simulink model "PSA_isa_velocity_control"  (R2020b)
settings: Solver=VariableStepAuto  StartTime=0.0  StopTime=40  RelTol=1e-3
values from neighbouring files (symbols this model uses):
  Kd = 1.2    [PSA_init.m]
  Kp = 1.5    [PSA_init.m]
  Lambda1 = 0.2    [PSA_init.m]
  tau1 = 0.7    [PSA_init.m]
undefined symbols (not defined in the file or in its folder): sigbuilder_block, x0
libraries: pid_lib x1
settings Model: Creator=anime  LastModifiedBy=anime

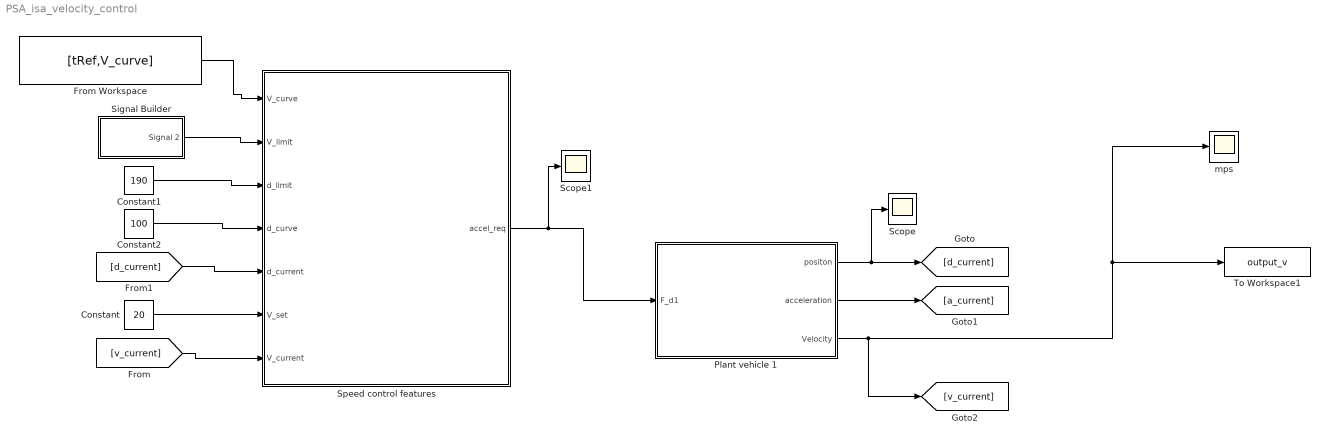
== system PSA_isa_velocity_control ==
  Constant : Constant  Value=20
  Constant1 : Constant  Value=190
  Constant2 : Constant  Value=100
  From Workspace : FromWorkspace  VariableName=[tRef,V_curve]  SampleTime=0.1
  Plant vehicle 1 : Subsystem
  Scope : Scope
  Scope1 : Scope
  Signal Builder : Subsystem  Tag=STV Subsys  LoadFcn=sigbuilder_block('load');  StartFcn=sigbuilder_block('start');  StopFcn=sigbuilder_block('stop');  ClipboardFcn=sigbuilder_block('clipboard');  mask(Sigbuilder block){tuvar=[0:10]}
      mask help: Simulink:masks:SigbuilderBlock_MD
      mask init:
      | if ~strcmp(get_param(bdroot(gcbh),'SimulationStatus'),'stopped') tuvar = sigbuilder_block('maskInit'); end
      settings: CopyFcn=sigbuilder_block('copy');  DeleteFcn=sigbuilder_block('delete');  ModelCloseFcn=sigbuilder_block('modelClose');  PreSaveFcn=sigbuilder_block('preSave');  PauseFcn=sigbuilder_block('pause');  ContinueFcn=sigbuilder_block('continue');  NameChangeFcn=sigbuilder_block('namechange');  OpenFcn=sigbuilder_block('open',[235.2 67.2 550.8 400.2 ]);  CloseFcn=sigbuilder_block('close');
      mask Display: plot(0, 0, 100, 100,[2, 2, 32, 32, 2], [68, 8, 8, 68, 68],[32, 2], [38, 38], [32, 19, 2],[53, 60, 44], [32, 17, 17, 2],[16, 16, 31, 31]);txt = getActiveGroup(gcbh);text(2, 100, txt,'verticalAlignment', 'top');
  Speed control features : Subsystem
  To Workspace1 : ToWorkspace  VariableName=output_v  SaveFormat=Timeseries  SampleTime=-1
  mps : Scope
  wires:
  Plant vehicle 1/3(Velocity) -> [v_current], mps/1, To Workspace1/1
  Plant vehicle 1/1(positon) -> Scope/1, [d_current]
  Plant vehicle 1/2(acceleration) -> [a_current]
  Speed control features/1(accel_req) -> Scope1/1, Plant vehicle 1/1(F_d1)
  [v_current] -> Speed control features/7(V_current)
  [d_current] -> Speed control features/5(d_current)
  Constant/1 -> Speed control features/6(V_set)
  Signal Builder/1(Signal 2) -> Speed control features/2(V_limit)
  Constant1/1 -> Speed control features/3("d_limit ")
  Constant2/1 -> Speed control features/4(d_curve)
  From Workspace/1 -> Speed control features/1(V_curve)

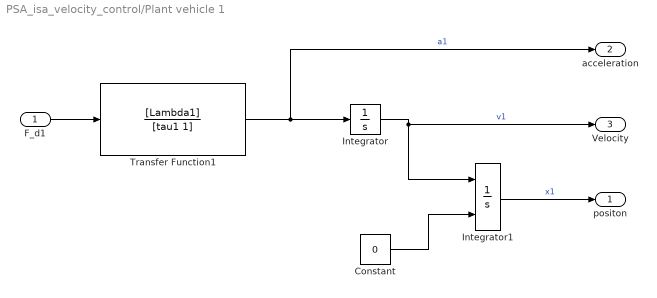
== system PSA_isa_velocity_control/Plant vehicle 1 ==
  F_d1 : Inport
  Constant : Constant  Value=0
  Integrator : Integrator  InitialCondition=3
  Integrator1 : Integrator  InitialConditionSource=external  InitialCondition=x0
  Transfer Function1 : TransferFcn  Numerator=[Lambda1]  Denominator=[tau1 1]
  positon : Outport
  acceleration : Outport  Port=2
  Velocity : Outport  Port=3
  wires:
  F_d1/1 -> Transfer Function1/1
  Transfer Function1/1 -> acceleration/1, Integrator/1  "a1"
  Integrator/1 -> Velocity/1, Integrator1/1  "v1"
  Constant/1 -> Integrator1/2
  Integrator1/1 -> positon/1  "x1"

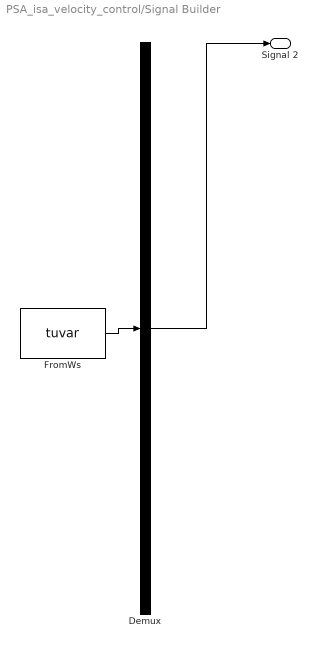
== system PSA_isa_velocity_control/Signal Builder ==
  Demux : Demux  Tag=STV Demux  Outputs=1
      settings: DisplayOption=none
  FromWs : FromWorkspace  Tag=STV FromWs  VariableName=tuvar
      SigBuilderData=|
      | common.afterFinalStr = 'Extrapolate'
      | common.sampleTime = 0
      | dataSet.timeRange = [0 40]
      | dataSet.name = 'Group 1'
      | sbobj.Groups.Name = 'Group 1'
      | sbobj.Groups.Signals.Name = 'Signal 2'
      | sbobj.Groups.Signals.XData = [0 25.2 25.2 40]
      | sbobj.Groups.Signals.YData = [11.11 11.11 16.667 16.667]
      | sbobj.Groups.TimeRange = [0 40]
  Signal 2 : Outport  Tag=STV Outport
  wires:
  FromWs/1 -> Demux/1
  Demux/1 -> Signal 2/1

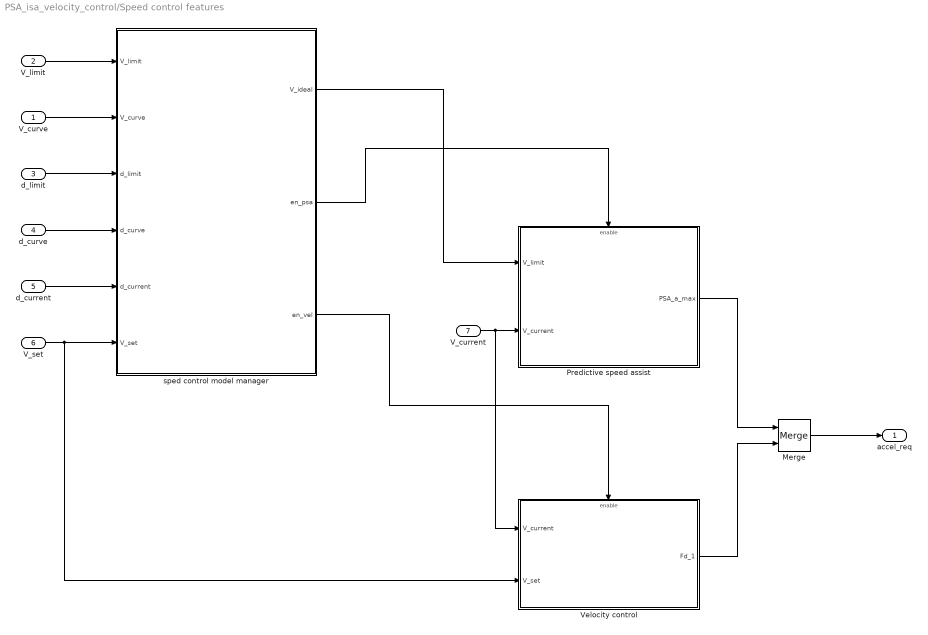
== system PSA_isa_velocity_control/Speed control features ==
  V_curve : Inport
  V_limit : Inport  Port=2
  "d_limit " : Inport  Port=3
  d_curve : Inport  Port=4
  d_current : Inport  Port=5
  V_set : Inport  Port=6
  V_current : Inport  Port=7
  Merge : Merge
  Predictive speed assist : Subsystem
  Velocity control : Subsystem
  sped control model manager : Subsystem
  accel_req : Outport
  wires:
  V_limit/1 -> sped control model manager/1(V_limit)
  "d_limit "/1 -> sped control model manager/3("d_limit ")
  d_curve/1 -> sped control model manager/4(d_curve)
  d_current/1 -> sped control model manager/5(d_current)
  V_set/1 -> Velocity control/2(V_set), sped control model manager/6(V_set)
  sped control model manager/3(en_vel) -> Velocity control/Enable
  sped control model manager/2(en_psa) -> Predictive speed assist/Enable
  sped control model manager/1(V_ideal) -> Predictive speed assist/1(V_limit)
  V_current/1 -> Velocity control/1(V_current), Predictive speed assist/2(V_current)
  Predictive speed assist/1(PSA_a_max) -> Merge/1
  Velocity control/1(Fd_1) -> Merge/2
  Merge/1 -> accel_req/1
  V_curve/1 -> sped control model manager/2(V_curve)

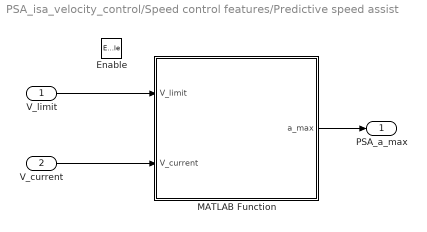
== system PSA_isa_velocity_control/Speed control features/Predictive speed assist ==
  V_limit : Inport
  V_current : Inport  Port=2
  Enable : EnablePort
  MATLAB Function : MATLAB Function  TreatAsAtomicUnit=on
  PSA_a_max : Outport
  wires:
  V_limit/1 -> MATLAB Function/1(V_limit)
  V_current/1 -> MATLAB Function/2(V_current)
  MATLAB Function/1(a_max) -> PSA_a_max/1

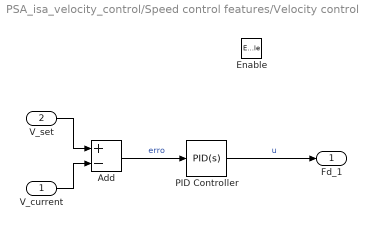
== system PSA_isa_velocity_control/Speed control features/Velocity control ==
  V_current : Inport
  V_set : Inport  Port=2
  Enable : EnablePort
  Add : Sum  Inputs=+-
  PID Controller : pid_lib/PID Controller  Controller=PID  Form=Parallel  TimeDomain=Continuous-time  UseExternalTs=off  SampleTime=-1  IntegratorMethod=Forward Euler  FilterMethod=Forward Euler  ControllerParametersSource=internal  P=Kp  I=0  D=Kd  UseFilter=on  N=100  TunerSelectOption=Transfer Function Based (PID Tuner App)  InitialConditionSource=internal  InitialConditionForIntegrator=0  InitialConditionForFilter=0  DifferentiatorICPrevScaledInput=0  ExternalReset=none  TrackingMode=off  Kt=1  LimitOutput=off  SatLimitsSource=internal  UpperSaturationLimit=inf  LowerSaturationLimit=-inf  LinearizeAsGain=on  AntiWindupMode=none  Kb=1  POutMin=[]  POutMax=[]  IOutMin=[]  IOutMax=[]  DOutMin=[]  DOutMax=[]  NOutMin=[]  NOutMax=[]  SumOutMin=[]  SumOutMax=[]  SaturationOutMin=[]  SaturationOutMax=[]  PParamMin=[]  PParamMax=[]  IParamMin=[]  IParamMax=[]  DParamMin=[]  DParamMax=[]  NParamMin=[]  NParamMax=[]  KbParamMin=[]  KbParamMax=[]  KtParamMin=[]  KtParamMax=[]  KbOutMin=[]  KbOutMax=[]  KtOutMin=[]  KtOutMax=[]  IntegratorOutMin=[]  IntegratorOutMax=[]  FilterOutMin=[]  FilterOutMax=[]  SumI1OutMin=[]  SumI1OutMax=[]  SumI2OutMin=[]  SumI2OutMax=[]  SumI3OutMin=[]  SumI3OutMax=[]  SumI4OutMin=[]  SumI4OutMax=[]  SumDOutMin=[]  SumDOutMax=[]  DifferentiatorOutMin=[]  DifferentiatorOutMax=[]  FilterDiffOutCoefMin=[]  FilterDiffOutCoefMax=[]  ReciprocalOutMin=[]  ReciprocalOutMax=[]  SumDenOutMin=[]  SumDenOutMax=[]  SumNumOutMin=[]  SumNumOutMax=[]  DivideOutMin=[]  DivideOutMax=[]  UdiffTsProdOutMin=[]  UdiffTsProdOutMax=[]  NTsProdOutMin=[]  NTsProdOutMax=[]  UintegralTsProdOutMin=[]  UintegralTsProdOutMax=[]  UngainTsProdOutMin=[]  UngainTsProdOutMax=[]  IntegratorContinuousStateAttributes=''  IntegratorStateMustResolveToSignalObject=off  IntegratorRTWStateStorageClass=Auto  FilterContinuousStateAttributes=''  FilterStateMustResolveToSignalObject=off  FilterRTWStateStorageClass=Auto  ParallelPVariant=InternalParameters  IdealPVariant=Disabled  IVariant=InternalParameters  DVariant=InternalParameters  IntegratorVariant=Continuous  SatVariant=Disabled  AWVariant=Passthrough  PCopyVariant=Disabled  TRVariant=Disabled  FdbkBlocksVariant=Forward  IdealPFdbkVariant=Disabled  SatFdbkVariant=Disabled  DerivativeFilterVariant=ContFilter  NVariant=InternalParameters  NCopyVariant=Disabled  FilterICVariant=InternalICsFilter  IntegratorICVariant=InternalICs  ExternalResetVariant=Disabled  TRSumVariant=Passthrough  SumFdbkVariant=Disabled  SumVariant=Sum_PID  TsampFilterVariant=InternalTs  TsampNgainVariant=Passthrough  TsampIntegralVariant=Passthrough  ExternalSaturationOutDataTypeStr=Inherit: Same as second input
  Fd_1 : Outport
  wires:
  PID Controller/1 -> Fd_1/1  "u"
  V_set/1 -> Add/1
  V_current/1 -> Add/2
  Add/1 -> PID Controller/1  "erro"

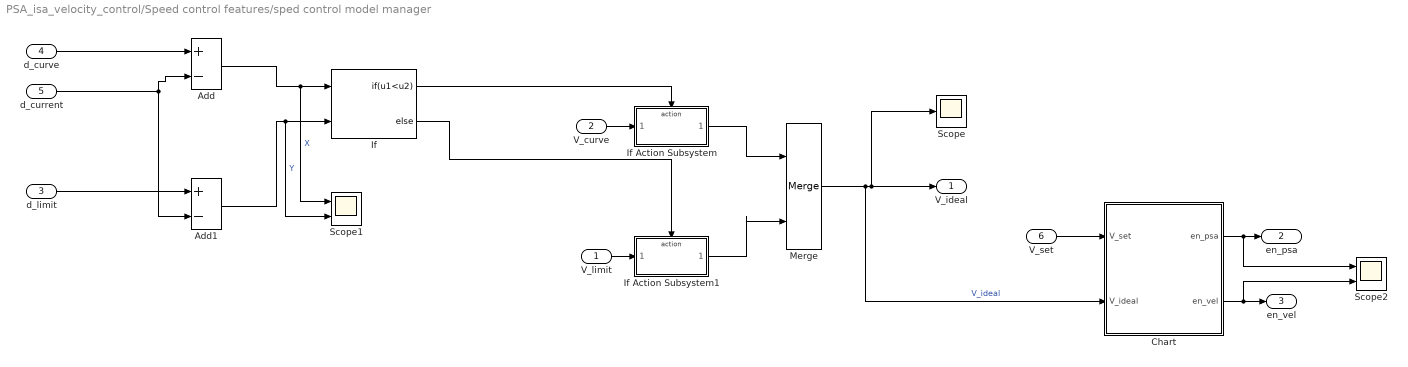
== system PSA_isa_velocity_control/Speed control features/sped control model manager ==
  V_limit : Inport
  V_curve : Inport  Port=2
  "d_limit " : Inport  Port=3
  d_curve : Inport  Port=4
  d_current : Inport  Port=5
  V_set : Inport  Port=6
  Add : Sum  Inputs=+-
  Add1 : Sum  Inputs=+-
  Chart : Stateflow chart  TreatAsAtomicUnit=on
  If : If  NumInputs=2  IfExpression=u1<u2
  If Action Subsystem : Subsystem  TreatAsAtomicUnit=on
  If Action Subsystem1 : Subsystem  TreatAsAtomicUnit=on
  Merge : Merge
  Scope : Scope
  Scope1 : Scope  NumInputPorts=2
  Scope2 : Scope  NumInputPorts=2
  V_ideal : Outport
  en_psa : Outport  Port=2
  en_vel : Outport  Port=3
  wires:
  d_current/1 -> Add/2, Add1/2
  d_curve/1 -> Add/1
  "d_limit "/1 -> Add1/1
  Add/1 -> Scope1/1, If/1  "X"
  Add1/1 -> Scope1/2, If/2  "Y"
  If/1 -> If Action Subsystem/Action
  If/2 -> If Action Subsystem1/Action
  If Action Subsystem/1(V_ideal) -> Merge/1
  If Action Subsystem1/1(V_ideal) -> Merge/2
  Merge/1 -> Chart/2(V_ideal), Scope/1, V_ideal/1  "V_ideal"
  V_set/1 -> Chart/1(V_set)
  Chart/1(en_psa) -> Scope2/1, en_psa/1
  Chart/2(en_vel) -> Scope2/2, en_vel/1
  V_curve/1 -> If Action Subsystem/1(V_curve)
  V_limit/1 -> If Action Subsystem1/1(V_curve)

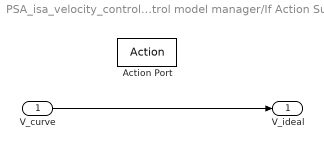
== system PSA_isa_velocity_control/Speed control features/sped control model manager/If Action Subsystem ==
  V_curve : Inport
  Action Port : ActionPort  ActionPortLabel=if(u1<u2)
  V_ideal : Outport
  wires:
  V_curve/1 -> V_ideal/1

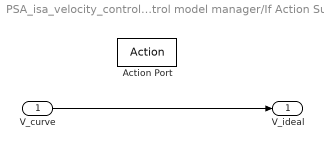
== system PSA_isa_velocity_control/Speed control features/sped control model manager/If Action Subsystem1 ==
  V_curve : Inport
  Action Port : ActionPort  ActionPortLabel=else
  V_ideal : Outport
  wires:
  V_curve/1 -> V_ideal/1

== matlab function PSA_isa_velocity_control/Speed control features/Predictive speed assist/MATLAB Function ==
  data: V_limit input; a_max output; V_current input
function a_max = PSA(V_limit,V_current)
if V_current < V_limit+0.2
    a_max = 2; % mpss
    
elseif V_current > V_limit+0.2
    a_max = -2; % mpss
else 
    a_max = 0;

end

== stateflow chart PSA_isa_velocity_control/Speed control features/sped control model manager/Chart ==
  state Velocity_control
    en:
    en_vel = true;
    en_psa = false;
  state PSA
    en:
    en_psa = true;
    en_vel = false;
  (default) -> Velocity_control
  Velocity_control -> PSA : [V_ideal < V_set]
  PSA -> Velocity_control : [V_ideal > V_set]
  data: en_psa output; en_vel output; V_set input; V_ideal input
